simulink model "task3_simulink"  (Simulink 7.3)
settings: Solver=ode45  StartTime=0.0  StopTime=10.0  RelTol=1e-3
libraries: simulink x3
settings Model: Creator=Natalia  LastModifiedBy=Natalia

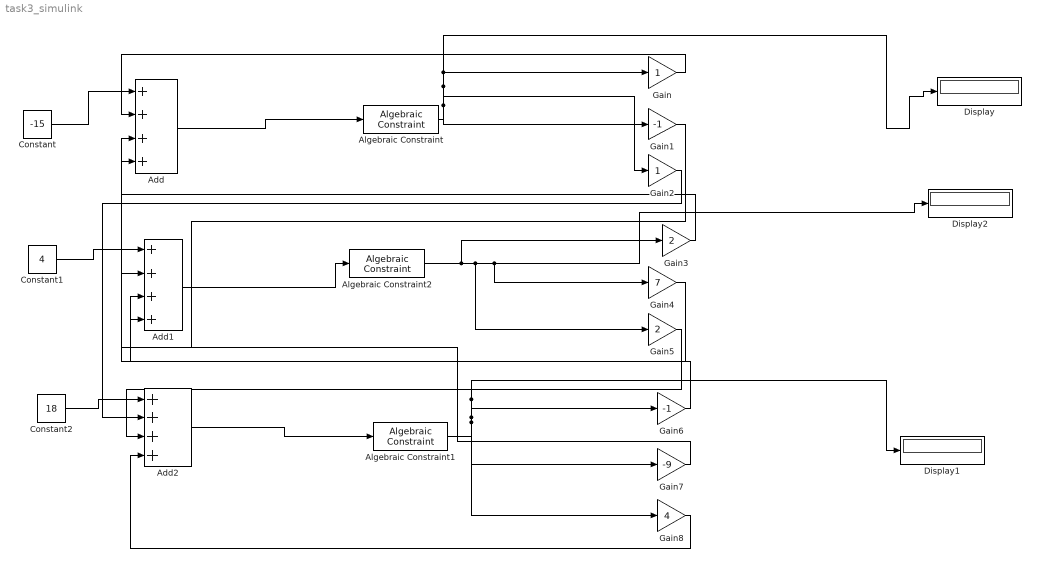
== system task3_simulink ==
  Add : Sum  Inputs=++++  OutDataType=fixdt(1, 16)  OutScaling=2^-10
  Add1 : Sum  Inputs=++++  OutDataType=fixdt(1, 16)  OutScaling=2^-10
  Add2 : Sum  Inputs=++++  OutDataType=fixdt(1, 16)  OutScaling=2^-10
  Algebraic Constraint : simulink/Math Operations/Algebraic Constraint  SystemSampleTime=-1  z0=0
  Algebraic Constraint1 : simulink/Math Operations/Algebraic Constraint  SystemSampleTime=-1  z0=0
  Algebraic Constraint2 : simulink/Math Operations/Algebraic Constraint  SystemSampleTime=-1  z0=0
  Constant : Constant  Value=-15  OutDataType=fixdt(1, 16)  OutScaling=2^0
  Constant1 : Constant  Value=4  OutDataType=fixdt(1, 16)  OutScaling=2^0
  Constant2 : Constant  Value=18  OutDataType=fixdt(1, 16)  OutScaling=2^0
  Display : Display
  Display1 : Display
  Display2 : Display
  Gain : Gain  ParameterDataType=fixdt(1, 16)  ParameterScaling=2^0  OutDataType=fixdt(1, 16)  OutScaling=2^0
  Gain1 : Gain  Gain=-1  ParameterDataType=fixdt(1, 16)  ParameterScaling=2^0  OutDataType=fixdt(1, 16)  OutScaling=2^0
  Gain2 : Gain  ParameterDataType=fixdt(1, 16)  ParameterScaling=2^0  OutDataType=fixdt(1, 16)  OutScaling=2^0
  Gain3 : Gain  Gain=2  ParameterDataType=fixdt(1, 16)  ParameterScaling=2^0  OutDataType=fixdt(1, 16)  OutScaling=2^0
  Gain4 : Gain  Gain=7  ParameterDataType=fixdt(1, 16)  ParameterScaling=2^0  OutDataType=fixdt(1, 16)  OutScaling=2^0
  Gain5 : Gain  Gain=2  ParameterDataType=fixdt(1, 16)  ParameterScaling=2^0  OutDataType=fixdt(1, 16)  OutScaling=2^0
  Gain6 : Gain  Gain=-1  ParameterDataType=fixdt(1, 16)  ParameterScaling=2^0  OutDataType=fixdt(1, 16)  OutScaling=2^0
  Gain7 : Gain  Gain=-9  ParameterDataType=fixdt(1, 16)  ParameterScaling=2^0  OutDataType=fixdt(1, 16)  OutScaling=2^0
  Gain8 : Gain  Gain=4  ParameterDataType=fixdt(1, 16)  ParameterScaling=2^0  OutDataType=fixdt(1, 16)  OutScaling=2^0
  wires:
  Constant/1 -> Add/1
  Constant1/1 -> Add1/1
  Constant2/1 -> Add2/1
  Add/1 -> Algebraic Constraint/1
  Algebraic Constraint/1 -> Gain/1, Display/1, Gain1/1, Gain2/1
  Gain/1 -> Add/2
  Gain1/1 -> Add1/2
  Gain2/1 -> Add2/2
  Add1/1 -> Algebraic Constraint2/1
  Add2/1 -> Algebraic Constraint1/1
  Algebraic Constraint2/1 -> Gain3/1, Display2/1, Gain4/1, Gain5/1
  Algebraic Constraint1/1 -> Display1/1, Gain6/1, Gain7/1, Gain8/1
  Gain3/1 -> Add/3
  Gain4/1 -> Add1/3
  Gain5/1 -> Add2/3
  Gain6/1 -> Add/4
  Gain7/1 -> Add1/4
  Gain8/1 -> Add2/4
